simulink model "ToyC"  (Simulink 9.2)
settings: Solver=ode45  StartTime=0.0  StopTime=10  RelTol=1e-3  EnableMultiTasking=on
libraries: simulink x1
settings Model: Creator=Luan Nguyen  LastModifiedBy=LuanNguyen
settings OptimizationCC: ExpressionDepthLimit=2147483647
settings DebuggingCC: MultiTaskDSMMsg=warning  MultiTaskCondExecSysMsg=none  FcnCallInpInsideContextMsg=error
settings GRTTargetCC: CombineOutputUpdateFcns=on  GRTInterface=off
settings ConfigComp: CovSFcnEnable=off

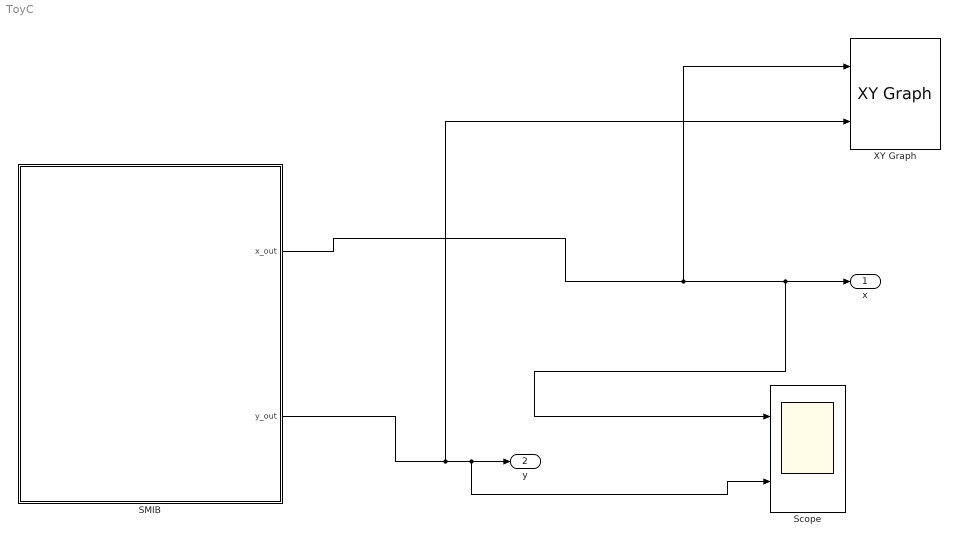
== system ToyC ==
  SMIB : Stateflow chart  TreatAsAtomicUnit=on
  Scope : Scope  NumInputPorts=2
  XY Graph : simulink/Sinks/XY Graph  xmin=-5  xmax=15  ymin=-5  ymax=10  st=-1
  x : Outport
  y : Outport  Port=2
  wires:
  SMIB/1(x_out) -> XY Graph/1, Scope/1, x/1
  SMIB/2(y_out) -> XY Graph/2, Scope/2, y/1

== stateflow chart SMIB ==
  settings: updateMethod=CONTINUOUS
  state Plant_1
    du:
    y_dot = 1;
    x_out = x;
    y_out = y;
  state Plant_2
    du:
    x_dot = 2;
    x_out = x;
    y_out = y;
  (default) -> Plant_1 : { x = 0; y = 0; }
  Plant_1 -> Plant_2 : [y> 5]
  Plant_2 -> Plant_2 : [x > 10]{x = 0;}
  data: x_out output double; y_out output double; x local double; y local double
  data x settings: updateMethod=SF_CONTINUOUS_TIME_DATA
  data y settings: updateMethod=SF_CONTINUOUS_TIME_DATA
